simulink model "untitled1"  (R2021a)
settings: Solver=VariableStepAuto  StartTime=0.0  StopTime=10.0  RelTol=1e-3
model workspace (MAT data in the model file):
  g = 9.8
  k = 4.8
  l = 4.9
libraries: simulink x1
settings Model: Creator=yyounes  LastModifiedBy=yyounes

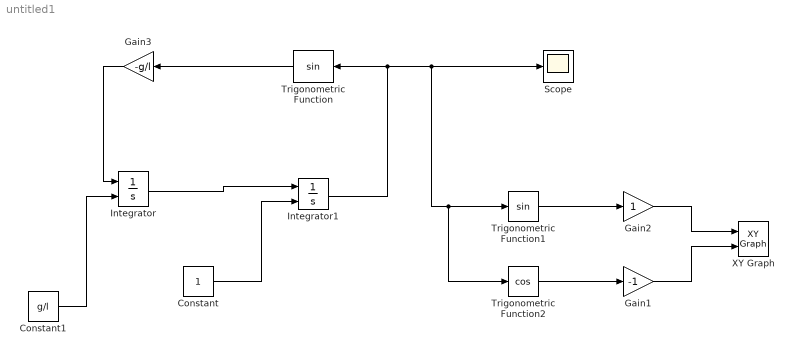
== system untitled1 ==
  Constant : Constant
  Constant1 : Constant  Value=g/l
  Gain1 : Gain  Gain=-1
  Gain2 : Gain
  Gain3 : Gain  Gain=-g/l
  Integrator : Integrator  InitialConditionSource=external
  Integrator1 : Integrator  InitialConditionSource=external
  Scope : Scope
  Trigonometric Function : Trigonometry
  Trigonometric Function1 : Trigonometry
  Trigonometric Function2 : Trigonometry  Operator=cos  ApproximationMethod=CORDIC
  XY Graph : simulink/Sinks/XY Graph  xmin=-1  xmax=1  ymin=-1  ymax=1  st=-1
  wires:
  Trigonometric Function/1 -> Gain3/1
  Integrator/1 -> Integrator1/1
  Gain3/1 -> Integrator/1
  Trigonometric Function1/1 -> Gain2/1
  Trigonometric Function2/1 -> Gain1/1
  Gain1/1 -> XY Graph/2
  Gain2/1 -> XY Graph/1
  Constant/1 -> Integrator1/2
  Integrator1/1 -> Trigonometric Function2/1, Trigonometric Function1/1, Scope/1, Trigonometric Function/1
  Constant1/1 -> Integrator/2
